simulink model "sim05"  (R2020a)
settings: Solver=VariableStepAuto  StartTime=0.0  StopTime=10.0  MaxStep=1/10  RelTol=1e-3
values from neighbouring files (symbols this model uses):
  du = 1    [lab05.m]
  u0 = 0    [lab05.m]
  w = Tabw(i)    [lab05.m]
  x0 = 0    [lab05.m]
  x10 = 0    [lab05.m]
settings Model: Creator=jakub  LastModifiedBy=jakub

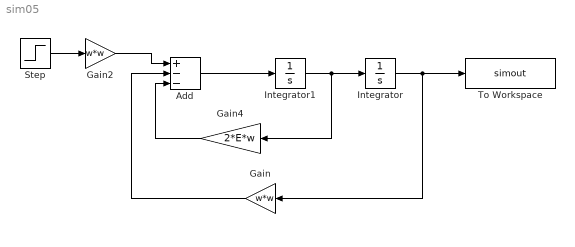
== system sim05 ==
  Add : Sum  Inputs=+--
  Gain : Gain  Gain=w*w
  Gain2 : Gain  Gain=w*w
  Gain4 : Gain  Gain=2*E*w
  Integrator : Integrator  InitialCondition=x0
  Integrator1 : Integrator  InitialCondition=x10
  Step : Step  Before=u0  After=u0+du  SampleTime=0
  To Workspace : ToWorkspace  VariableName=simout  SampleTime=-1
  wires:
  Integrator1/1 -> Gain4/1, Integrator/1
  Integrator/1 -> Gain/1, To Workspace/1
  Add/1 -> Integrator1/1
  Gain2/1 -> Add/1
  Step/1 -> Gain2/1
  Gain4/1 -> Add/3
  Gain/1 -> Add/2
